simulink model "controllerModel"  (R2022a)
settings: Solver=VariableStepAuto  StartTime=0.0  StopTime=inf  RelTol=1e-3
values from neighbouring files (symbols this model uses):
  A = B_full    [controllerInit.m]
  A_full = zeros(nX * (nH + 1), nX)    [controllerInit.m]
  D = -B_full' * Q_full    [controllerInit.m]
  F = B_full' * Q_full * A_full    [controllerInit.m]
  fCutoff = 8    [controllerInit.m]
  H = B_full' * Q_full * B_full + R_full    [controllerInit.m]
  lb_qp = lb_u_full    [controllerInit.m]
  lb_x_full = ub_x_full    [controllerInit.m]
  ref_struct = struct()    [controllerInit.m]    (also in ready_simulink_model.m)
  steerTorqLim = 3    [controllerInit.m]
  tracker_height = 0.9    [controllerInit.m]
  Ts_mpc = 1/80    (= 0.0125)    [controllerInit.m]
  Ts_ser = 1/200    (= 0.005)    [controllerInit.m]
  Ts_udp = 1/160    (= 0.00625)    [controllerInit.m]
  ub_qp = ub_u_full    [controllerInit.m]
  ub_x_full = zeros(nX * (nH + 1), 1)    [controllerInit.m]
undefined symbols (not defined in the file or in its folder): Serial_Port, Standard_Devices, UDP_Protocol
libraries: sldrtlib x5, simulink_extras x1, dspstat3 x1, sharedtransform x1
settings Model: Creator=simonas  LastModifiedBy=sudo
settings HardwareCC: ProdBitPerLong=64  ProdHWDeviceType=Intel->x86-64 (Linux 64)
settings RTWCC: Description=Simulink Desktop Real-Time  SystemTargetFile=sldrt.tlc  TemplateMakefile=sldrt.tmf  RTWCompilerOptimization=on
settings RTWCC: CustomInclude=|
  | C:\Users\sudo\Desktop\Simonas\qpOASES-releases-3.2.1\include
  | C:\Users\sudo\Desktop\Simonas\qpOASES-releases-3.2.1\interfaces\simulink
  | C:\Users\sudo\Desktop\Simonas\qpOASES-releases-3.2.1\src
settings CodeAppCC: MaxIdLength=95
settings SimulinkDesktopRealTimeCC: TargetLibSuffix=_sldrt.a  TargetPreCompLibLocation=C:\Program Files\MATLAB\R2022a\toolbox\sldrt\lib\win64

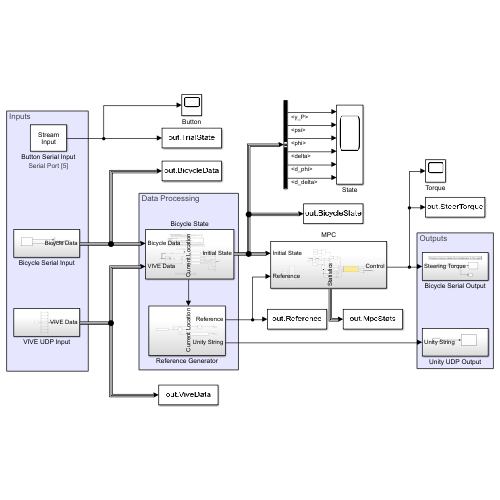
[thumbnail: Simulink's stored preview of the top-level diagram]
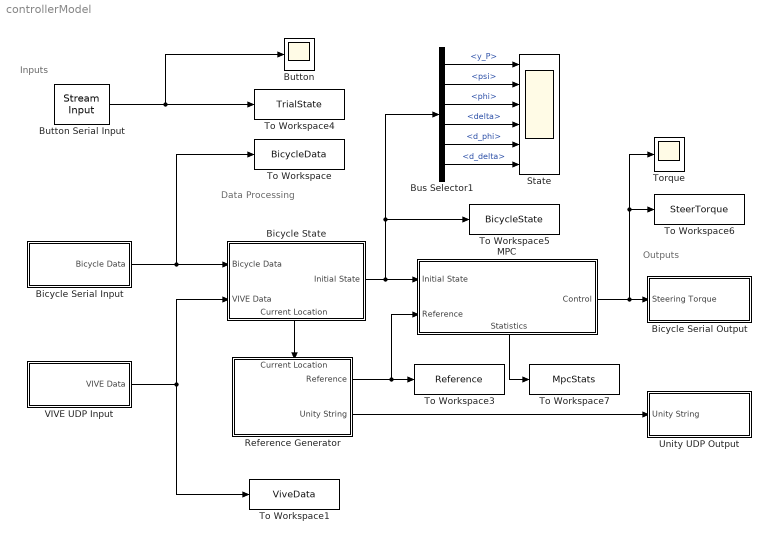
== system controllerModel ==
  note: Inputs
  note: Data Processing
  note: Outputs
  Bicycle Serial Input : Subsystem
  Bicycle Serial Output : Subsystem
  Bicycle State : Subsystem
      settings: PortSchema="{\"entries\":[{\"content\":{\"sides\":[{\"content\":{\"connectorIds\":[\"In1\",\"In2\"]},\"type\":\"ConnectorPlacement.EquallySpacedRectSide\",\"uuid\":\"c5d89f74-e35e-400b-a49a-6a7c3bbb3cee\"},{\"content\":{\"connectorIds\":[\"Out1\"],\"side\":\"RIGHT\"},\"type\":\"ConnectorPlacement.EquallySpacedRectSide\",\"uuid\":\"d3946c1d-493c-4283-9feb-9c130facb0a9\"},{\"content\":{\"connectorIds\":[],\"side\":\"TOP\"},\"type\":\"ConnectorPlacement.EquallySpacedRectSide\",\"uuid\":\"f7eeef6e-15d0-4138-b893-66df70237323\"},{\"content\":{\"connectorIds\":[\"Out2\"],\"side\":\"BOTTOM\"},\"type\":\"ConnectorPlacement.EquallySpacedRectSide\",\"uuid\":\"d8cc5cfa-3fb7-476d-9b2c-860b356f327e\"}]},\"type\":\"ConnectorPlacement.EquallySpacedConnector\",\"uuid\":\"85360968-76db-44cc-98f9-7355ff2a9269\"}],\"packageUris\":[\"http://schema.mathworks.com/mf0/Connector/R2020b\"],\"version\":\"1.0\"}"
  Bus Selector1 : BusSelector  OutputSignals=y_P,psi,phi,delta,d_phi,d_delta
  Button : Scope
  Button Serial Input : sldrtlib/Stream Input  SampleTime=0.05  MaxMissedTicks=1000000  ShowMissedTicks=off  YieldWhenWaiting=off  DrvName=Standard_Devices/Serial_Port  DrvAddress=5  DrvOptions=[115200 8 0 0 0 0 0 0]  DataTypes='int32'  FormatString='%d'  Terminator={'\n', '\r'}  ShowReady=off  ShowError=off
      settings: AttributesFormatString=Serial Port [5]  SourceProductBaseCode=WT
  MPC : Subsystem
      settings: PortSchema="{\"entries\":[{\"content\":{\"sides\":[{\"content\":{\"connectorIds\":[\"In1\",\"In2\"]},\"type\":\"ConnectorPlacement.EquallySpacedRectSide\",\"uuid\":\"837940b0-492f-49e7-ad78-2f53a96cfdb0\"},{\"content\":{\"connectorIds\":[\"Out1\"],\"side\":\"RIGHT\"},\"type\":\"ConnectorPlacement.EquallySpacedRectSide\",\"uuid\":\"0b454771-57c7-4798-97e4-6e41a25b36dc\"},{\"content\":{\"connectorIds\":[],\"side\":\"TOP\"},\"type\":\"ConnectorPlacement.EquallySpacedRectSide\",\"uuid\":\"d0d77e63-f0c6-441e-9a4a-b6dfb0057ad2\"},{\"content\":{\"connectorIds\":[\"Out2\"],\"side\":\"BOTTOM\"},\"type\":\"ConnectorPlacement.EquallySpacedRectSide\",\"uuid\":\"b6921f02-8dc3-4ff1-8cb0-61ac83bc5ab1\"}]},\"type\":\"ConnectorPlacement.EquallySpacedConnector\",\"uuid\":\"6905a0a5-9fd3-4ab9-9143-61679843e617\"}],\"packageUris\":[\"http://schema.mathworks.com/mf0/Connector/R2020b\"],\"version\":\"1.0\"}"
  Reference Generator : Subsystem
      settings: PortSchema="{\"entries\":[{\"content\":{\"sides\":[{\"content\":{\"connectorIds\":[]},\"type\":\"ConnectorPlacement.EquallySpacedRectSide\",\"uuid\":\"995dcb62-78f8-423c-99d5-aa9c538d86ef\"},{\"content\":{\"connectorIds\":[\"Out1\",\"Out2\"],\"side\":\"RIGHT\"},\"type\":\"ConnectorPlacement.EquallySpacedRectSide\",\"uuid\":\"d6e446ff-77b4-4bca-8c68-e505a29969fe\"},{\"content\":{\"connectorIds\":[\"In1\"],\"side\":\"TOP\"},\"type\":\"ConnectorPlacement.EquallySpacedRectSide\",\"uuid\":\"a2ee3f9a-5385-4b4c-abf0-7e00a59d14cf\"}]},\"type\":\"ConnectorPlacement.EquallySpacedConnector\",\"uuid\":\"6b026230-ac01-4f6d-82d7-753dc9fb2975\"}],\"packageUris\":[\"http://schema.mathworks.com/mf0/Connector/R2020b\"],\"version\":\"1.0\"}"
  State : Scope  NumInputPorts=6
  To Workspace : ToWorkspace  VariableName=BicycleData  SaveFormat=Timeseries  SampleTime=-1
  To Workspace1 : ToWorkspace  VariableName=ViveData  SaveFormat=Timeseries  SampleTime=-1
  To Workspace3 : ToWorkspace  VariableName=Reference  SaveFormat=Timeseries  SampleTime=-1
  To Workspace4 : ToWorkspace  VariableName=TrialState  SaveFormat=Structure With Time  SampleTime=-1
  To Workspace5 : ToWorkspace  VariableName=BicycleState  SaveFormat=Timeseries  SampleTime=-1
  To Workspace6 : ToWorkspace  VariableName=SteerTorque  SaveFormat=Timeseries  SampleTime=-1
  To Workspace7 : ToWorkspace  VariableName=MpcStats  SaveFormat=Timeseries  SampleTime=-1
  Torque : Scope
  Unity UDP Output : Subsystem
  VIVE UDP Input : Subsystem
  wires:
  Button Serial Input/1 -> Button/1, To Workspace4/1
  Bicycle State/2(Current Location) -> Reference Generator/1(Current Location)
  Bicycle Serial Input/1(Bicycle Data) -> To Workspace/1, Bicycle State/1(Bicycle Data)
  VIVE UDP Input/1(VIVE Data) -> Bicycle State/2(VIVE Data), To Workspace1/1
  Bicycle State/1(Initial State) -> MPC/1(Initial State), Bus Selector1/1, To Workspace5/1
  Reference Generator/1(Reference) -> MPC/2(Reference), To Workspace3/1
  MPC/1(Control) -> To Workspace6/1, Torque/1, Bicycle Serial Output/1(Steering Torque)
  Reference Generator/2(Unity String) -> Unity UDP Output/1(Unity String)
  MPC/2(Statistics) -> To Workspace7/1
  Bus Selector1/6 -> State/6  "<d_delta>"
  Bus Selector1/2 -> State/2  "<psi>"
  Bus Selector1/1 -> State/1  "<y_P>"
  Bus Selector1/3 -> State/3  "<phi>"
  Bus Selector1/4 -> State/4  "<delta>"
  Bus Selector1/5 -> State/5  "<d_phi>"

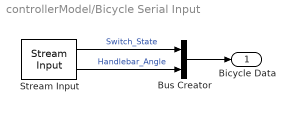
== system controllerModel/Bicycle Serial Input ==
  Bus Creator : BusCreator  Inputs=2
  Stream Input : sldrtlib/Stream Input  SampleTime=Ts_ser  MaxMissedTicks=1000000  ShowMissedTicks=off  YieldWhenWaiting=on  DrvName=Standard_Devices/Serial_Port  DrvAddress=6  DrvOptions=[115200 8 0 0 0 0 0 0]  DataTypes={'uint8','double'}  FormatString='%d,%f'  Terminator={'\n'}  ShowReady=off  ShowError=off
      settings: AttributesFormatString=Serial Port [6]  SourceProductBaseCode=WT
  Bicycle Data : Outport
  wires:
  Stream Input/1 -> Bus Creator/1  "Switch_State"
  Stream Input/2 -> Bus Creator/2  "Handlebar_Angle"
  Bus Creator/1 -> Bicycle Data/1

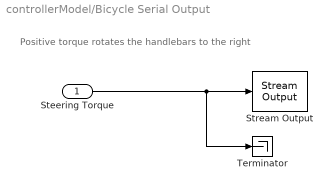
== system controllerModel/Bicycle Serial Output ==
  note: Positive torque rotates the handlebars to the right
  Steering Torque : Inport
  Stream Output : sldrtlib/Stream Output  SampleTime=Ts_mpc  MaxMissedTicks=1000000  ShowMissedTicks=off  YieldWhenWaiting=on  DrvName=Standard_Devices/Serial_Port  DrvAddress=6  DrvOptions=[115200 8 0 0 0 0 0 0]  PortSizes=1  FormatString='%.3f\n'  ShowReady=off  ShowError=off  InitialValue=[]  FinalValue=[]
      settings: AttributesFormatString=Serial Port [6]  SourceProductBaseCode=WT
  Terminator : Terminator
  wires:
  Steering Torque/1 -> Stream Output/1, Terminator/1

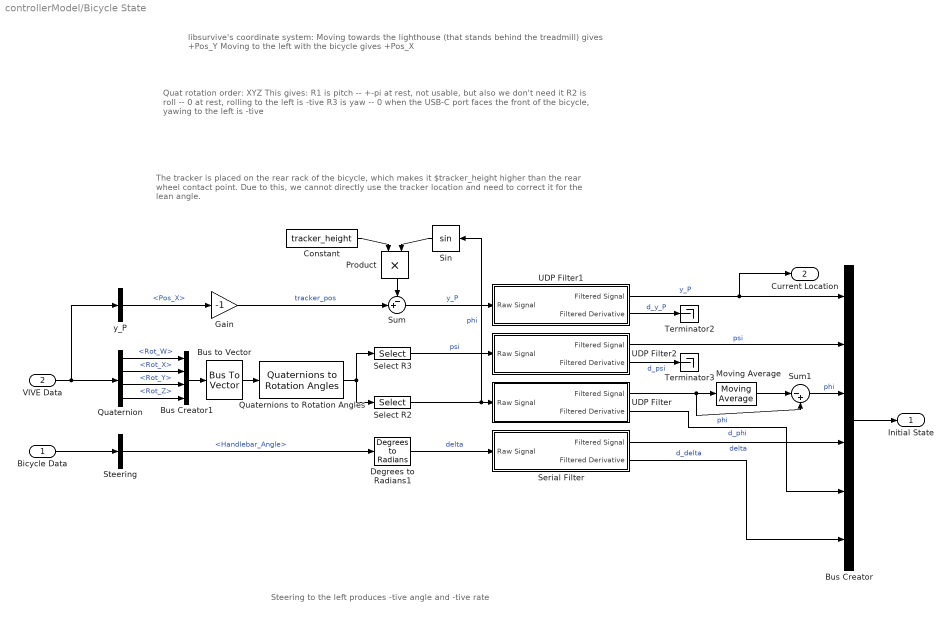
== system controllerModel/Bicycle State ==
  note: The tracker is placed on the rear rack of the bicycle, which makes it $tracker_height higher than the rear wheel contact point. Due to this, we cannot directly use the tracker location and need to correct it for the lean angle.
  note: Steering to the left produces -tive angle and -tive rate
  note: libsurvive's coordinate system:
      | Moving towards the lighthouse (that stands behind the treadmill) gives +Pos_Y
      | Moving to the left with the bicycle gives +Pos_X
  note: Quat rotation order: XYZ
      | This gives:
      | R1 is pitch -- +-pi at rest, not usable, but also we don't need it
      | R2 is roll -- 0 at rest, rolling to the left is -tive
      | R3 is yaw -- 0 when the USB-C port faces the front of the bicycle, yawing to the left is -tive
  Bicycle Data : Inport
  VIVE Data : Inport  Port=2
  Bus Creator : BusCreator  Inputs=6
  Bus Creator1 : BusCreator  Inputs=4
  Bus to Vector : BusToVector
  Constant : Constant  Value=tracker_height
  Degrees to Radians1 : simulink_extras/Transformations/Degrees to Radians
  Gain : Gain  Gain=-1
  Moving Average : dspstat3/Moving Average  Method=Sliding window  ForgettingFactorPort=off  SpecifyWindowLength=on  WindowLength=5/Ts_udp  ForgettingFactor=0.9  SimulateUsing=Code generation
  Product : Product
  Quaternion : BusSelector  OutputSignals=Rot_W,Rot_X,Rot_Y,Rot_Z
  Quaternions to Rotation Angles : sharedtransform/Quaternions to Rotation Angles  rotationOrder=XYZ  aMode=aMode
      settings: SourceProductBaseCode=AE,PW,DR,MT,VE
  Select R2 : Selector  InputPortWidth=3  IndexOptions=Index vector (dialog)  Indices=2  OutputSizes=1
  Select R3 : Selector  InputPortWidth=3  IndexOptions=Index vector (dialog)  Indices=3  OutputSizes=1
  Serial Filter : Subsystem
  Sin : Trigonometry
  Steering : BusSelector  OutputSignals=Handlebar_Angle
  Sum : Sum  Inputs=-+|
  Sum1 : Sum  Inputs=|-+
  Terminator2 : Terminator
  Terminator3 : Terminator
  UDP Filter : Subsystem
  UDP Filter1 : Subsystem
  UDP Filter2 : Subsystem
  y_P : BusSelector  OutputSignals=Pos_X
  Initial State : Outport
  Current Location : Outport  Port=2
  wires:
  VIVE Data/1 -> y_P/1, Quaternion/1
  Quaternion/2 -> Bus Creator1/2  "<Rot_X>"
  Quaternion/3 -> Bus Creator1/3  "<Rot_Y>"
  Quaternion/4 -> Bus Creator1/4  "<Rot_Z>"
  Select R2/1 -> UDP Filter/1(Raw Signal), Sin/1  "phi"
  y_P/1 -> Gain/1  "<Pos_X>"
  Bicycle Data/1 -> Steering/1
  Steering/1 -> Degrees to Radians1/1  "<Handlebar_Angle>"
  Bus Creator/1 -> Initial State/1
  Quaternion/1 -> Bus Creator1/1  "<Rot_W>"
  Bus Creator1/1 -> Bus to Vector/1
  Bus to Vector/1 -> Quaternions to Rotation Angles/1
  Quaternions to Rotation Angles/1 -> Select R3/1, Select R2/1
  Degrees to Radians1/1 -> Serial Filter/1(Raw Signal)  "delta"
  Gain/1 -> Sum/2  "tracker_pos"
  Product/1 -> Sum/1
  Constant/1 -> Product/1
  Sin/1 -> Product/2
  UDP Filter/1(Filtered Signal) -> Sum1/2, Moving Average/1  "phi"
  UDP Filter/2(Filtered Derivative) -> Bus Creator/5  "d_phi"
  Serial Filter/1(Filtered Signal) -> Bus Creator/4  "delta"
  Serial Filter/2(Filtered Derivative) -> Bus Creator/6  "d_delta"
  Sum/1 -> UDP Filter1/1(Raw Signal)  "y_P"
  UDP Filter1/1(Filtered Signal) -> Bus Creator/1, Current Location/1  "y_P"
  UDP Filter1/2(Filtered Derivative) -> Terminator2/1  "d_y_P"
  Select R3/1 -> UDP Filter2/1(Raw Signal)  "psi"
  UDP Filter2/1(Filtered Signal) -> Bus Creator/2  "psi"
  UDP Filter2/2(Filtered Derivative) -> Terminator3/1  "d_psi"
  Moving Average/1 -> Sum1/1
  Sum1/1 -> Bus Creator/3  "phi"

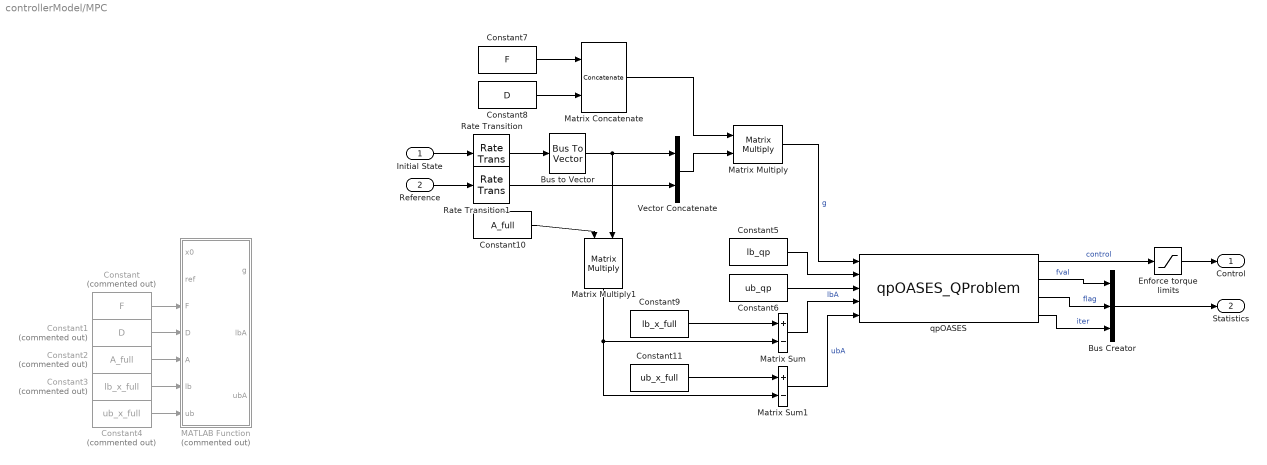
== system controllerModel/MPC ==
  Initial State : Inport
  Reference : Inport  Port=2
  Bus Creator : BusCreator  Inputs=3
  Bus to Vector : BusToVector
  Constant : Constant  Commented=on  Value=F  VectorParams1D=off  SampleTime=Ts_mpc
  Constant1 : Constant  Commented=on  Value=D  VectorParams1D=off  SampleTime=Ts_mpc
  Constant10 : Constant  Value=A_full  VectorParams1D=off  SampleTime=Ts_mpc
  Constant11 : Constant  Value=ub_x_full  VectorParams1D=off  SampleTime=Ts_mpc
  Constant2 : Constant  Commented=on  Value=A_full  VectorParams1D=off  SampleTime=Ts_mpc
  Constant3 : Constant  Commented=on  Value=lb_x_full  VectorParams1D=off  SampleTime=Ts_mpc
  Constant4 : Constant  Commented=on  Value=ub_x_full  VectorParams1D=off  SampleTime=Ts_mpc
  Constant5 : Constant  Value=lb_qp  VectorParams1D=off  SampleTime=Ts_mpc
  Constant6 : Constant  Value=ub_qp  VectorParams1D=off  SampleTime=Ts_mpc
  Constant7 : Constant  Value=F  VectorParams1D=off  SampleTime=Ts_mpc
  Constant8 : Constant  Value=D  VectorParams1D=off  SampleTime=Ts_mpc
  Constant9 : Constant  Value=lb_x_full  VectorParams1D=off  SampleTime=Ts_mpc
  Enforce torque limits : Saturate  UpperLimit=steerTorqLim  LowerLimit=-steerTorqLim
  MATLAB Function : MATLAB Function  Commented=on  TreatAsAtomicUnit=on
  Matrix Concatenate : Concatenate  Mode=Multidimensional array  ConcatenateDimension=2
  Matrix Sum : Sum  Inputs=+-
  Matrix Sum1 : Sum  Inputs=+-
  Matrix Multiply : Product  Multiplication=Matrix(*)
  Matrix Multiply1 : Product  Multiplication=Matrix(*)
  Rate Transition : RateTransition  Deterministic=off  OutPortSampleTime=Ts_mpc
  Rate Transition1 : RateTransition  OutPortSampleTime=Ts_mpc
  Vector Concatenate : Concatenate
  qpOASES : S-Function  FunctionName=qpOASES_QProblem  Parameters=H,A  SFunctionDeploymentMode=off  EnableBusSupport=off
  Control : Outport
  Statistics : Outport  Port=2
  wires:
  Constant5/1 -> qpOASES/2
  Constant/1 -> MATLAB Function/3(F)
  Constant1/1 -> MATLAB Function/4(D)
  Initial State/1 -> Rate Transition/1
  Constant4/1 -> MATLAB Function/7(ub)
  Constant3/1 -> MATLAB Function/6(lb)
  Constant6/1 -> qpOASES/3
  qpOASES/4 -> Bus Creator/3  "iter"
  qpOASES/2 -> Bus Creator/1  "fval"
  Constant2/1 -> MATLAB Function/5(A)
  Reference/1 -> Rate Transition1/1
  qpOASES/3 -> Bus Creator/2  "flag"
  qpOASES/1 -> Enforce torque limits/1  "control"
  Bus Creator/1 -> Statistics/1
  Enforce torque limits/1 -> Control/1
  Constant7/1 -> Matrix Concatenate/1
  Constant8/1 -> Matrix Concatenate/2
  Bus to Vector/1 -> Matrix Multiply1/2, Vector Concatenate/1
  Matrix Concatenate/1 -> Matrix Multiply/1
  Vector Concatenate/1 -> Matrix Multiply/2
  Matrix Multiply/1 -> qpOASES/1  "g"
  Constant9/1 -> Matrix Sum/1
  Constant10/1 -> Matrix Multiply1/1
  Matrix Multiply1/1 -> Matrix Sum1/2, Matrix Sum/2
  Constant11/1 -> Matrix Sum1/1
  Matrix Sum/1 -> qpOASES/4  "lbA"
  Matrix Sum1/1 -> qpOASES/5  "ubA"
  Rate Transition/1 -> Bus to Vector/1
  Rate Transition1/1 -> Vector Concatenate/2

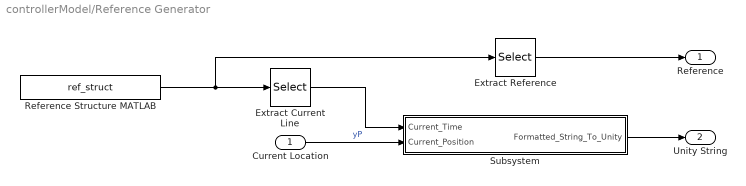
== system controllerModel/Reference Generator ==
  Current Location : Inport
  Extract Current Line : Selector  InputPortWidth=size(ref_struct.signals.values, 2)  IndexOptions=Index vector (dialog)  Indices=1  OutputSizes=1
  Extract Reference : Selector  InputPortWidth=size(ref_struct.signals.values, 2)  IndexOptions=Index vector (dialog)  Indices=2:size(ref_struct.signals.values, 2)  OutputSizes=1
  Reference Structure MATLAB : FromWorkspace  VariableName=ref_struct  SampleTime=Ts_mpc  Interpolate=off  ZeroCross=off  OutputAfterFinalValue=Cyclic repetition
  Subsystem : Subsystem
  Reference : Outport
  Unity String : Outport  Port=2  OutDataTypeStr=string
  wires:
  Subsystem/1(Formatted_String_To_Unity) -> Unity String/1
  Reference Structure MATLAB/1 -> Extract Reference/1, Extract Current Line/1
  Extract Current Line/1 -> Subsystem/1(Current_Time)
  Extract Reference/1 -> Reference/1
  Current Location/1 -> Subsystem/2(Current_Position)  "yP"

== system controllerModel/Unity UDP Output ==
  Unity String : Inport
  Stream Output : sldrtlib/Stream Output  SampleTime=Ts_udp  MaxMissedTicks=1000000  ShowMissedTicks=off  YieldWhenWaiting=on  DrvName=Standard_Devices/UDP_Protocol  DrvAddress=8005  DrvOptions=[0 8006 49 50 55 46 48 46 48 46 49 0 0 0 0 0 0 0 0 0 0 0 0 0 0 0 0 0 0 0 0 0 0 0 0 0 0 0 0 0 0 0 0 0 0 0 0 0 0 0 0 0 0 0 0 0 0 0 0 0 0 0 0 0 0 0 0 0 0 0 0 0 0 0 0 0 0 0 0 0 0 0 0 0 0 0 0 0 0 0 0 0 0 0 0 0 0 0 0 0 0 0 0 0 0 0 0 0 0 0 0 0 0 0 0 0 0 0 0 0 0 0 0 0 0 0 0 0 0 0 0 0 0 0 0 0 0 0 0 0 0 0 0 0 0 0 0 0 0 0 0 0 0 0 0 0 0 0 0 0 0 0 0 0 0 0 0 0 0 0 0 0 0 0 0 0 0 0 0 0 0 0 0 0 0 0 0 0 0 0 0 0 0 0 0 0 0 0 0 0 0 0 0 0 0 0 0 0 0 0 0 0 0 0 0 0 0 0 0 0 0 0 0 0 0 0 0 0 0 0 0 0 0 0 0 0 0 0 0 0 0 0 0 0 0 0 0 0 0 0 0 0 0 0 0 0]  PortSizes=1  FormatString='%s'  ShowReady=off  ShowError=off  InitialValue=[]  FinalValue=[]
      settings: AttributesFormatString=UDP Protocol [8005]  SourceProductBaseCode=WT
  wires:
  Unity String/1 -> Stream Output/1

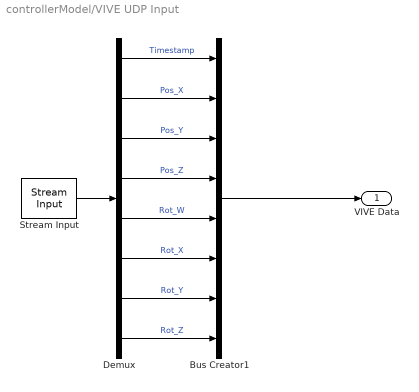
== system controllerModel/VIVE UDP Input ==
  Bus Creator1 : BusCreator  Inputs=8
  Demux : Demux  Outputs=8
  Stream Input : sldrtlib/Stream Input  SampleTime=Ts_udp  MaxMissedTicks=1000000  ShowMissedTicks=off  YieldWhenWaiting=on  DrvName=Standard_Devices/UDP_Protocol  DrvAddress=4950  DrvOptions=[0 16385 0 0 0 0 0 0 0 0 0 0 0 0 0 0 0 0 0 0 0 0 0 0 0 0 0 0 0 0 0 0 0 0 0 0 0 0 0 0 0 0 0 0 0 0 0 0 0 0 0 0 0 0 0 0 0 0 0 0 0 0 0 0 0 0 0 0 0 0 0 0 0 0 0 0 0 0 0 0 0 0 0 0 0 0 0 0 0 0 0 0 0 0 0 0 0 0 0 0 0 0 0 0 0 0 0 0 0 0 0 0 0 0 0 0 0 0 0 0 0 0 0 0 0 0 0 0 0 0 0 0 0 0 0 0 0 0 0 0 0 0 0 0 0 0 0 0 0 0 0 0 0 0 0 0 0 0 0 0 0 0 0 0 0 0 0 0 0 0 0 0 0 0 0 0 0 0 0 0 0 0 0 0 0 0 0 0 0 0 0 0 0 0 0 0 0 0 0 0 0 0 0 0 0 0 0 0 0 0 0 0 0 0 0 0 0 0 0 0 0 0 0 0 0 0 0 0 0 0 0 0 0 0 0 0 0 0 0 0 0 0 0 0 0 0 0 0 0 0 0 0 0 0 0 0]  DataTypes={'8*double'}  FormatString='%f,%f,%f,%f,%f,%f,%f,%f'  Terminator='\n'  ShowReady=off  ShowError=off
      settings: AttributesFormatString=UDP Protocol [4950]  SourceProductBaseCode=WT
  VIVE Data : Outport
  wires:
  Demux/4 -> Bus Creator1/4  "Pos_Z"
  Demux/5 -> Bus Creator1/5  "Rot_W"
  Demux/7 -> Bus Creator1/7  "Rot_Y"
  Demux/6 -> Bus Creator1/6  "Rot_X"
  Demux/1 -> Bus Creator1/1  "Timestamp"
  Demux/2 -> Bus Creator1/2  "Pos_X"
  Demux/8 -> Bus Creator1/8  "Rot_Z"
  Demux/3 -> Bus Creator1/3  "Pos_Y"
  Bus Creator1/1 -> VIVE Data/1
  Stream Input/1 -> Demux/1

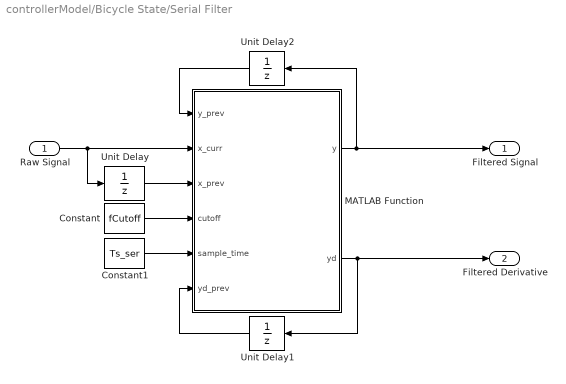
== system controllerModel/Bicycle State/Serial Filter ==
  Raw Signal : Inport
  Constant : Constant  Value=fCutoff  SampleTime=Ts_ser
  Constant1 : Constant  Value=Ts_ser  SampleTime=Ts_ser
  MATLAB Function : MATLAB Function  TreatAsAtomicUnit=on
  Unit Delay : UnitDelay  SampleTime=Ts_ser  HasFrameUpgradeWarning=on
  Unit Delay1 : UnitDelay  SampleTime=Ts_ser  HasFrameUpgradeWarning=on
  Unit Delay2 : UnitDelay  SampleTime=Ts_ser  HasFrameUpgradeWarning=on
  Filtered Signal : Outport
  Filtered Derivative : Outport  Port=2
  wires:
  MATLAB Function/1(y) -> Unit Delay2/1, Filtered Signal/1
  MATLAB Function/2(yd) -> Unit Delay1/1, Filtered Derivative/1
  Raw Signal/1 -> Unit Delay/1, MATLAB Function/2(x_curr)
  Unit Delay/1 -> MATLAB Function/3(x_prev)
  Constant/1 -> MATLAB Function/4(cutoff)
  Constant1/1 -> MATLAB Function/5(sample_time)
  Unit Delay2/1 -> MATLAB Function/1(y_prev)
  Unit Delay1/1 -> MATLAB Function/6(yd_prev)

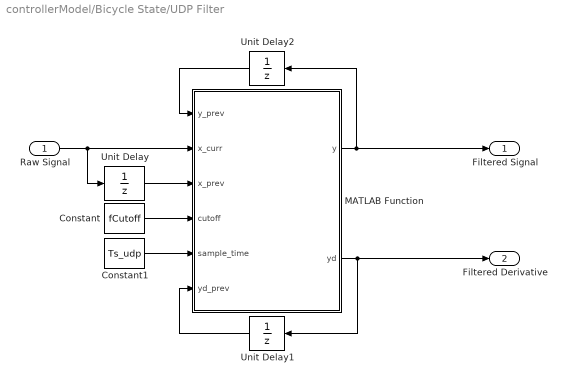
== system controllerModel/Bicycle State/UDP Filter ==
  Raw Signal : Inport
  Constant : Constant  Value=fCutoff  SampleTime=Ts_udp
  Constant1 : Constant  Value=Ts_udp  SampleTime=Ts_udp
  MATLAB Function : MATLAB Function  TreatAsAtomicUnit=on
  Unit Delay : UnitDelay  SampleTime=Ts_udp  HasFrameUpgradeWarning=on
  Unit Delay1 : UnitDelay  SampleTime=Ts_udp  HasFrameUpgradeWarning=on
  Unit Delay2 : UnitDelay  SampleTime=Ts_udp  HasFrameUpgradeWarning=on
  Filtered Signal : Outport
  Filtered Derivative : Outport  Port=2
  wires:
  MATLAB Function/1(y) -> Unit Delay2/1, Filtered Signal/1
  MATLAB Function/2(yd) -> Unit Delay1/1, Filtered Derivative/1
  Raw Signal/1 -> Unit Delay/1, MATLAB Function/2(x_curr)
  Unit Delay/1 -> MATLAB Function/3(x_prev)
  Constant/1 -> MATLAB Function/4(cutoff)
  Constant1/1 -> MATLAB Function/5(sample_time)
  Unit Delay2/1 -> MATLAB Function/1(y_prev)
  Unit Delay1/1 -> MATLAB Function/6(yd_prev)

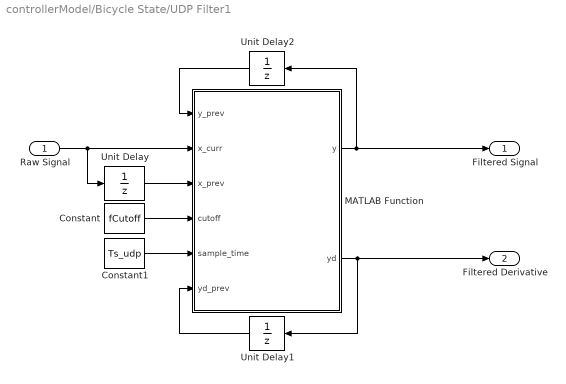
== system controllerModel/Bicycle State/UDP Filter1 ==
  Raw Signal : Inport
  Constant : Constant  Value=fCutoff  SampleTime=Ts_udp
  Constant1 : Constant  Value=Ts_udp  SampleTime=Ts_udp
  MATLAB Function : MATLAB Function  TreatAsAtomicUnit=on
  Unit Delay : UnitDelay  SampleTime=Ts_udp  HasFrameUpgradeWarning=on
  Unit Delay1 : UnitDelay  SampleTime=Ts_udp  HasFrameUpgradeWarning=on
  Unit Delay2 : UnitDelay  SampleTime=Ts_udp  HasFrameUpgradeWarning=on
  Filtered Signal : Outport
  Filtered Derivative : Outport  Port=2
  wires:
  MATLAB Function/1(y) -> Unit Delay2/1, Filtered Signal/1
  MATLAB Function/2(yd) -> Unit Delay1/1, Filtered Derivative/1
  Raw Signal/1 -> Unit Delay/1, MATLAB Function/2(x_curr)
  Unit Delay/1 -> MATLAB Function/3(x_prev)
  Constant/1 -> MATLAB Function/4(cutoff)
  Constant1/1 -> MATLAB Function/5(sample_time)
  Unit Delay2/1 -> MATLAB Function/1(y_prev)
  Unit Delay1/1 -> MATLAB Function/6(yd_prev)

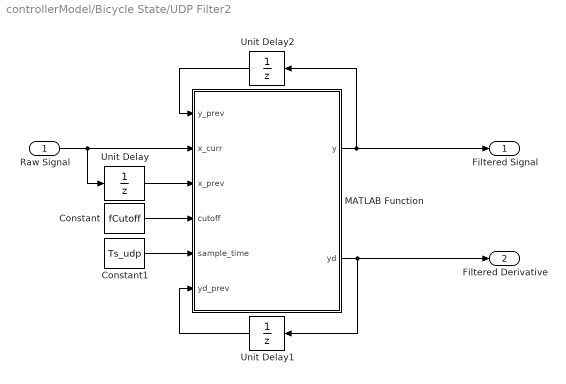
== system controllerModel/Bicycle State/UDP Filter2 ==
  Raw Signal : Inport
  Constant : Constant  Value=fCutoff  SampleTime=Ts_udp
  Constant1 : Constant  Value=Ts_udp  SampleTime=Ts_udp
  MATLAB Function : MATLAB Function  TreatAsAtomicUnit=on
  Unit Delay : UnitDelay  SampleTime=Ts_udp  HasFrameUpgradeWarning=on
  Unit Delay1 : UnitDelay  SampleTime=Ts_udp  HasFrameUpgradeWarning=on
  Unit Delay2 : UnitDelay  SampleTime=Ts_udp  HasFrameUpgradeWarning=on
  Filtered Signal : Outport
  Filtered Derivative : Outport  Port=2
  wires:
  MATLAB Function/1(y) -> Unit Delay2/1, Filtered Signal/1
  MATLAB Function/2(yd) -> Unit Delay1/1, Filtered Derivative/1
  Raw Signal/1 -> Unit Delay/1, MATLAB Function/2(x_curr)
  Unit Delay/1 -> MATLAB Function/3(x_prev)
  Constant/1 -> MATLAB Function/4(cutoff)
  Constant1/1 -> MATLAB Function/5(sample_time)
  Unit Delay2/1 -> MATLAB Function/1(y_prev)
  Unit Delay1/1 -> MATLAB Function/6(yd_prev)

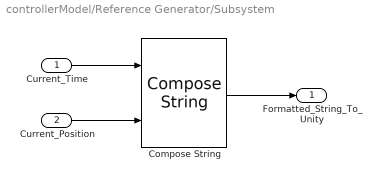
== system controllerModel/Reference Generator/Subsystem ==
  Current_Time : Inport
  Current_Position : Inport  Port=2
  Compose String : ComposeString  Format="\"%.0f,%.3f\\n\""
  Formatted_String_To_Unity : Outport
  wires:
  Current_Position/1 -> Compose String/2
  Compose String/1 -> Formatted_String_To_Unity/1
  Current_Time/1 -> Compose String/1

== matlab function controllerModel/Bicycle State/UDP Filter/MATLAB Function ==
  data: y_prev input; y output; x_curr input; x_prev input; cutoff input; sample_time input; yd_prev input; yd output
function [y, yd] = realtime_filter(y_prev, x_curr, x_prev, ...
                                   cutoff, sample_time, yd_prev)
a = (2*pi * cutoff^2);
b = sqrt(2) * 2*pi * cutoff;
h = sample_time;
denom = 4 + 2*h*b + h^2*a;

A = (4 + 2*h*b - h^2*a) / denom;
B = 4*h / denom;
C = -4*h*a / denom;
D = (4 - 2*h*b - h^2*a) / denom;
E = 2*h^2*a / denom;
F = 4*h*a / denom;

y = A * y_prev + B * yd_prev + E * (x_curr + x_prev) / 2;
yd = C * y_prev + D * yd_prev + F * (x_curr + x_prev) / 2;

== matlab function controllerModel/MPC/MATLAB Function ==
  data: g output; x0 input; lbA output; ref input; F input; D input; A input; lb input; ub input; ubA output
function [g, lbA, ubA] = findOnlineQP(x0, ref, F, D, A, lb, ub)

lbA = lb - A * x0;
ubA = ub - A * x0;
g = [F, D] * [x0; ref];

== matlab function controllerModel/Bicycle State/Serial Filter/MATLAB Function ==
  data: y_prev input; y output; x_curr input; x_prev input; cutoff input; sample_time input; yd_prev input; yd output
function [y, yd] = realtime_filter(y_prev, x_curr, x_prev, ...
                                   cutoff, sample_time, yd_prev)
a = (2*pi * cutoff^2);
b = sqrt(2) * 2*pi * cutoff;
h = sample_time;
denom = 4 + 2*h*b + h^2*a;

A = (4 + 2*h*b - h^2*a) / denom;
B = 4*h / denom;
C = -4*h*a / denom;
D = (4 - 2*h*b - h^2*a) / denom;
E = 2*h^2*a / denom;
F = 4*h*a / denom;

y = A * y_prev + B * yd_prev + E * (x_curr + x_prev) / 2;
yd = C * y_prev + D * yd_prev + F * (x_curr + x_prev) / 2;

== matlab function controllerModel/Bicycle State/UDP Filter1/MATLAB Function ==
  data: y_prev input; y output; x_curr input; x_prev input; cutoff input; sample_time input; yd_prev input; yd output
function [y, yd] = realtime_filter(y_prev, x_curr, x_prev, ...
                                   cutoff, sample_time, yd_prev)
a = (2*pi * cutoff^2);
b = sqrt(2) * 2*pi * cutoff;
h = sample_time;
denom = 4 + 2*h*b + h^2*a;

A = (4 + 2*h*b - h^2*a) / denom;
B = 4*h / denom;
C = -4*h*a / denom;
D = (4 - 2*h*b - h^2*a) / denom;
E = 2*h^2*a / denom;
F = 4*h*a / denom;

y = A * y_prev + B * yd_prev + E * (x_curr + x_prev) / 2;
yd = C * y_prev + D * yd_prev + F * (x_curr + x_prev) / 2;

== matlab function controllerModel/Bicycle State/UDP Filter2/MATLAB Function ==
  data: y_prev input; y output; x_curr input; x_prev input; cutoff input; sample_time input; yd_prev input; yd output
function [y, yd] = realtime_filter(y_prev, x_curr, x_prev, ...
                                   cutoff, sample_time, yd_prev)
a = (2*pi * cutoff^2);
b = sqrt(2) * 2*pi * cutoff;
h = sample_time;
denom = 4 + 2*h*b + h^2*a;

A = (4 + 2*h*b - h^2*a) / denom;
B = 4*h / denom;
C = -4*h*a / denom;
D = (4 - 2*h*b - h^2*a) / denom;
E = 2*h^2*a / denom;
F = 4*h*a / denom;

y = A * y_prev + B * yd_prev + E * (x_curr + x_prev) / 2;
yd = C * y_prev + D * yd_prev + F * (x_curr + x_prev) / 2;
